simulink model "s_akalm1"  (Simulink 4.00)
settings: Solver=ode45  SolverMode=SingleTasking  StartTime=0.0  StopTime=100  FixedStep=0.1  RelTol=1e-3  AbsTol=1e-6
values from neighbouring files (symbols this model uses):
  Ap = prozess_ss.a    [akalm1.m]
  As = stoerung_ss.a    [akalm1.m]
  Bp = prozess_ss.b    [akalm1.m]
  Bs = stoerung_ss.b    [akalm1.m]
  Cp = prozess_ss.c    [akalm1.m]
  Cs = stoerung_ss.c    [akalm1.m]
  Dp = prozess_ss.d    [akalm1.m]
  Ds = stoerung_ss.d    [akalm1.m]
  min_step = 0.05    [abeob1.m]    (also in akalm1.m = 0.1; alqr1.m = 0.1; alqrd1.m = 0.1; apol1.m = 0.1)
  qm = 0.01    [akalm1.m]
  qp = 0.01    [akalm1.m]
  Ts = 0.5    [abeob1.m]    (also in akalm1.m = 0.25; alqrd1.m = 0.25; kalm2.m; kalm3.m)
settings Model: LastModifiedBy=Administrator  SaveTime=off  SaveOutput=off  LimitDataPoints=off  BlockReductionOpt=off

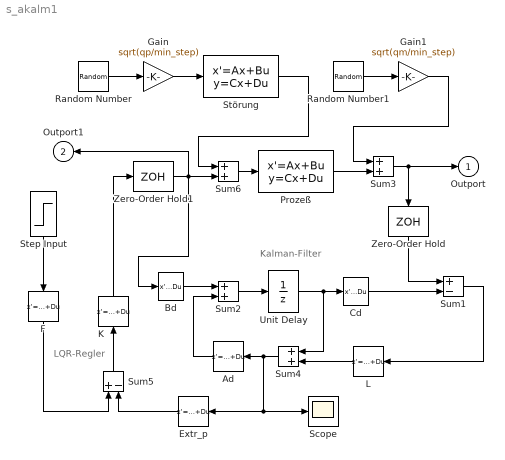
== system s_akalm1 ==
  note: Kalman-Filter
  note: LQR-Regler
  Ad : StateSpace  Orientation=left  A=[]  B=[]  C=[]  D=K  X0=0  Realization=auto  AbsoluteTolerance=auto  mask(Matrix Gain){@1=Ad}
      mask prompts: @1 "Gain matrix:"
      mask help: Matrix Gain.
      mask init:
      | K = @1;
      mask Help: Multiplies input vector by entered matrix to produce output vector (y=Au).
      mask Display: disp('K')
  Bd : StateSpace  A=[]  B=[]  C=[]  D=K  X0=0  Realization=auto  AbsoluteTolerance=auto  mask(Matrix Gain){@1=Bd}
      mask prompts: @1 "Gain matrix:"
      mask help: Matrix Gain.
      mask init:
      | K = @1;
      mask Help: Multiplies input vector by entered matrix to produce output vector (y=Au).
      mask Display: disp('K')
  Cd : StateSpace  A=[]  B=[]  C=[]  D=K  X0=0  Realization=auto  AbsoluteTolerance=auto  mask(Matrix Gain){@1=Cd}
      mask prompts: @1 "Gain matrix:"
      mask help: Matrix Gain.
      mask init:
      | K = @1;
      mask Help: Multiplies input vector by entered matrix to produce output vector (y=Au).
      mask Display: disp('K')
  Extr_p : StateSpace  Orientation=left  A=[]  B=[]  C=[]  D=K  X0=0  Realization=auto  AbsoluteTolerance=auto  mask(Matrix Gain){@1=Extr_p}
      mask prompts: @1 "Gain matrix:"
      mask help: Matrix Gain.
      mask init:
      | K = @1;
      mask Help: Multiplies input vector by entered matrix to produce output vector (y=Au).
      mask Display: disp('K')
  F : StateSpace  Orientation=down  A=[]  B=[]  C=[]  D=K  X0=0  Realization=auto  AbsoluteTolerance=auto  mask(Matrix Gain){@1=F}
      mask prompts: @1 "Gain matrix:"
      mask help: Matrix Gain.
      mask init:
      | K = @1;
      mask Help: Multiplies input vector by entered matrix to produce output vector (y=Au).
      mask Display: disp('K')
  Gain : Gain  Gain=sqrt(qp/min_step)  Multiplication=Element-wise(K.*u)  SaturateOnIntegerOverflow=on
  Gain1 : Gain  Gain=sqrt(qm/min_step)  Multiplication=Element-wise(K.*u)  SaturateOnIntegerOverflow=on
  K : StateSpace  Orientation=up  A=[]  B=[]  C=[]  D=K  X0=0  Realization=auto  AbsoluteTolerance=auto  mask(Matrix Gain){@1=K}
      mask prompts: @1 "Gain matrix:"
      mask help: Matrix Gain.
      mask init:
      | K = @1;
      mask Help: Multiplies input vector by entered matrix to produce output vector (y=Au).
      mask Display: disp('K')
  L : StateSpace  Orientation=left  A=[]  B=[]  C=[]  D=K  X0=0  Realization=auto  AbsoluteTolerance=auto  mask(Matrix Gain){@1=L}
      mask prompts: @1 "Gain matrix:"
      mask help: Matrix Gain.
      mask init:
      | K = @1;
      mask Help: Multiplies input vector by entered matrix to produce output vector (y=Au).
      mask Display: disp('K')
  Prozeß : StateSpace  A=Ap  B=Bp  C=Cp  D=Dp  X0=0  Realization=auto  AbsoluteTolerance=auto
  Random Number : RandomNumber  Mean=0  Variance=1  Seed=0  SampleTime=0
  Random Number1 : RandomNumber  Mean=0  Variance=1  Seed=0  SampleTime=0
  Scope : Scope
      settings: TickLabels=on  TimeRange=100.000000  YMin=-10.000000  YMax=10.000000  SaveToWorkspace=off  SaveName=ScopeData  DataFormat=Array  LimitDataPoints=on  MaxDataPoints=5000
  Step Input : Step  Orientation=down  Time=2.5  Before=0  After=1  SampleTime=0
  Störung : StateSpace  A=As  B=Bs  C=Cs  D=Ds  X0=0  Realization=auto  AbsoluteTolerance=auto
  Sum1 : Sum  Inputs=+-  SaturateOnIntegerOverflow=on
  Sum2 : Sum  Inputs=++  SaturateOnIntegerOverflow=on
  Sum3 : Sum  Inputs=++  SaturateOnIntegerOverflow=on
  Sum4 : Sum  Orientation=left  Inputs=++  SaturateOnIntegerOverflow=on
  Sum5 : Sum  Orientation=up  Inputs=+-  SaturateOnIntegerOverflow=on
  Sum6 : Sum  Inputs=++  SaturateOnIntegerOverflow=on
  Unit Delay : UnitDelay  X0=0  SampleTime=Ts
  Zero-Order Hold : ZeroOrderHold  Orientation=down  SampleTime=Ts
  Zero-Order Hold1 : ZeroOrderHold  SampleTime=Ts
  Outport : Outport  Port=1  InitialOutput=0
  Outport1 : Outport  Orientation=left  Port=2  InitialOutput=0
  wires:
  Sum3/1 -> Zero-Order Hold/1, Outport/1
  Störung/1 -> Sum6/1
  Zero-Order Hold1/1 -> Outport1/1, Sum6/2, Bd/1
  Sum6/1 -> Prozeß/1
  Extr_p/1 -> Sum5/2
  Sum4/1 -> Scope/1, Extr_p/1, Ad/1
  Gain1/1 -> Sum3/1
  Prozeß/1 -> Sum3/2
  F/1 -> Sum5/1
  Step Input/1 -> F/1
  Sum5/1 -> K/1
  K/1 -> Zero-Order Hold1/1
  Sum1/1 -> L/1
  L/1 -> Sum4/2
  Unit Delay/1 -> Sum4/1, Cd/1
  Ad/1 -> Sum2/2
  Bd/1 -> Sum2/1
  Sum2/1 -> Unit Delay/1
  Cd/1 -> Sum1/2
  Zero-Order Hold/1 -> Sum1/1
  Gain/1 -> Störung/1
  Random Number/1 -> Gain/1
  Random Number1/1 -> Gain1/1
